simulink model "EfestoRocketEngine_28_04_23"  (R2023a)
settings: Solver=VariableStepAuto  StartTime=0.0  StopTime=50  RelTol=1e-3
libraries: matrix_library x2, shared3dof x1
settings Model: Creator=giuse  LastModifiedBy=mattiasaba
settings DebuggingCC: UnconnectedInputMsg=warning  UnconnectedOutputMsg=warning  UnconnectedLineMsg=warning
settings ModelReferenceCC: EnableRefExpFcnMdlSchedulingChecks=on
settings RTWCC: DLArmComputeVersion=19.05

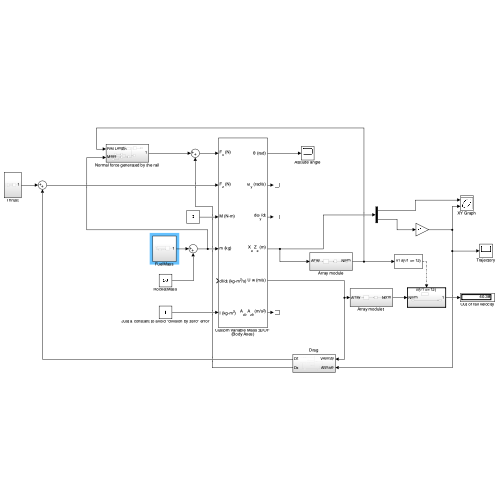
[thumbnail: Simulink's stored preview of the top-level diagram]
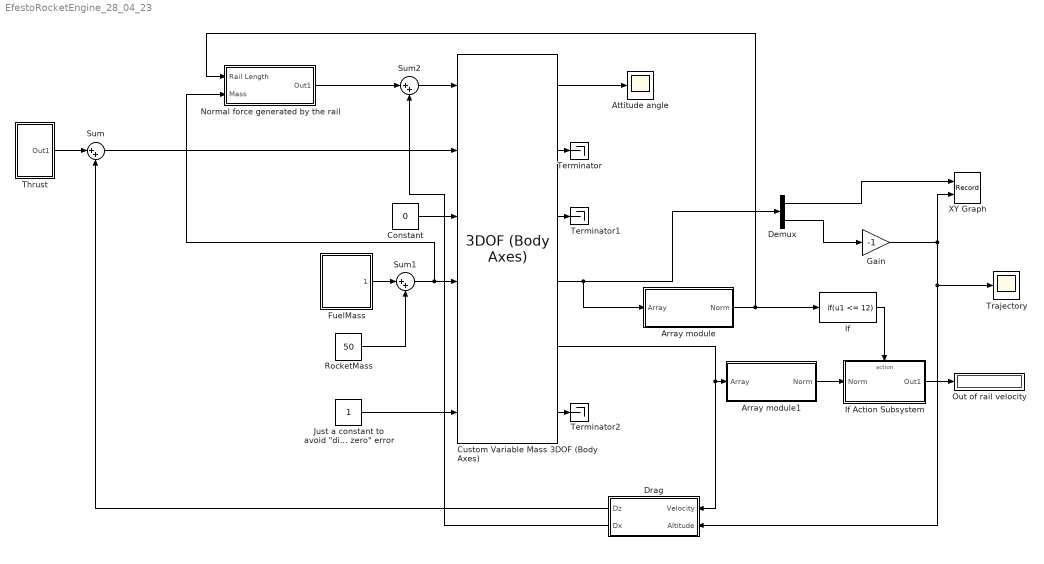
== system EfestoRocketEngine_28_04_23 ==
  Array module : Subsystem
  Array module1 : Subsystem
  Attitude angle : Scope
  Constant : Constant  Value=0
  Custom Variable Mass 3DOF (Body Axes) : shared3dof/3DOF (Body Axes)  units=Metric (MKS)  mtype=Custom Variable  v_ini=0  theta_ini=pi  alpha_ini=0  pos_ini=[0 0]  q_ini=0  mass=1.0  mass_e=0.5  mass_f=3.0  Iyy=1.0  Iyy_e=0.5  Iyy_f=3.0  g_in=Internal  g=9.81  vre_flag=off  abi_flag=off  aMode=0  vel_statename=''  theta_statename=''  pos_statename=''  q_statename=''  mass_statename=''
  Demux : Demux  Outputs=2
  Drag : Subsystem
  FuelMass : Subsystem
  Gain : Gain  Gain=-1
  If : If  IfExpression=u1 <= 12  ShowElse=off
  If Action Subsystem : Subsystem  TreatAsAtomicUnit=on
  "Just a constant to avoid \"division by zero\" error" : Constant
  Normal force generated by the rail : Subsystem
  Out of rail velocity : Display
  RocketMass : Constant  Value=50
  Sum : Sum  Inputs=|++
  Sum1 : Sum  Inputs=|++
  Sum2 : Sum  Inputs=|++
  Terminator : Terminator
  Terminator1 : Terminator
  Terminator2 : Terminator
  Thrust : Subsystem
  Trajectory : Scope
  XY Graph : Record  FileSettingsInternal="{\"entries\":[{\"content\":{\"excelSettings\":{\"content\":{},\"type\":\"Streamout.ExcelSettings\"}},\"type\":\"Streamout.FileSettingStorage\",\"uuid\":\"102b2f02-9d14-4766-8d69-63aa978f5510\"}],\"packageUris\":[\"http://schema.mathworks.com/mf0/streamout_blocks/R2020a\"],\"version\":\"1.0\"}"  Layout=[1 1]  SignalsInternal="{\"entries\":[{\"content\":{\"signals\":[{\"content\":{\"blockPath\":[\"EfestoRocketEngine_28_04_23/XY Graph\"],\"dimensions\":[1],\"domain\":\"EfestoRocketEngine_28_04_23/XY Graph\",\"lineColor\":\"#a2142f\",\"plots\":[1],\"port\":1,\"sid\":[\"\"],\"signalID\":96,\"signalName\":\"Demux:1\"},\"type\":\"RecordBlkView.Signal\",\"uuid\":\"11d17661-1dd1-4241-8cf8-6f9b05c222c4\"},{\"content\":{\"blockPath\":[\"EfestoRocketEngine_28_04_23/XY Graph\"],\"dimensions\":[1],\"domain\":\"EfestoRocketEngine_28_04_23/XY Graph\",\"lineColor\":\"#139fff\",\"plots\":[1],\"port\":2,\"sid\":[\"\"],\"signalID\":100,\"signalName\":\"Gain\"},\"type\":\"RecordBlkView.Signal\",\"uuid\":\"dbca8d71-ba0e-47b5-92a1-924a943d85be\"}]},\"type\":\"RecordBlkView.InputSignals\",\"uuid\":\"7a493edc-8874-4727-801b-36ee9696f784\"}],\"packageUris\":[\"http://schema.mathworks.com/mf0/streamout_blocks/R2020a\"],\"version\":\"1.0\"}"  VisualizationBindings="{\"xyplotplugin\":{\"info\":[{\"series\":[{\"bindingParametersList\":[{\"parameter\":\"X-Axis\",\"signalID\":96,\"signalName\":\"Demux:1\"},{\"parameter\":\"Y-Axis\",\"signalID\":100,\"signalName\":\"Gain\"}],\"seriesID\":31883}],\"subplotID\":1}]}}"  CompatibilityTag=XY  st=-1
  wires:
  Gain/1 -> Drag/2(Altitude), Trajectory/1, XY Graph/2
  Demux/2 -> Gain/1
  Demux/1 -> XY Graph/1
  Custom Variable Mass 3DOF (Body Axes)/4 -> Array module/1(Array), Demux/1
  Custom Variable Mass 3DOF (Body Axes)/5 -> Drag/1(Velocity), Array module1/1(Array)
  Drag/1(Dz) -> Sum/2
  Custom Variable Mass 3DOF (Body Axes)/1 -> Attitude angle/1
  Constant/1 -> Custom Variable Mass 3DOF (Body Axes)/3
  Custom Variable Mass 3DOF (Body Axes)/2 -> Terminator/1
  Custom Variable Mass 3DOF (Body Axes)/3 -> Terminator1/1
  Custom Variable Mass 3DOF (Body Axes)/6 -> Terminator2/1
  RocketMass/1 -> Sum1/2
  "Just a constant to avoid \"division by zero\" error"/1 -> Custom Variable Mass 3DOF (Body Axes)/6
  If/1 -> If Action Subsystem/Action
  If Action Subsystem/1(Out1) -> Out of rail velocity/1
  Sum/1 -> Custom Variable Mass 3DOF (Body Axes)/2
  Sum1/1 -> Normal force generated by the rail/2(Mass), Custom Variable Mass 3DOF (Body Axes)/4
  Array module1/1(Norm) -> If Action Subsystem/1(Norm)
  Array module/1(Norm) -> Normal force generated by the rail/1(Rail Length), If/1
  Normal force generated by the rail/1(Out1) -> Sum2/1
  FuelMass/1(1) -> Sum1/1
  Thrust/1(Out1) -> Sum/1
  Drag/2(Dx) -> Sum2/2
  Sum2/1 -> Custom Variable Mass 3DOF (Body Axes)/1

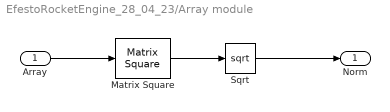
== system EfestoRocketEngine_28_04_23/Array module ==
  Array : Inport
  Matrix Square : matrix_library/Matrix Square  OutMin=[]  OutMax=[]
      settings: LibrarySourceBlock=|
      | simulink/Matrix
      | Operations/Matrix
      | Square
  Sqrt : Sqrt
  Norm : Outport
  wires:
  Array/1 -> Matrix Square/1
  Matrix Square/1 -> Sqrt/1
  Sqrt/1 -> Norm/1

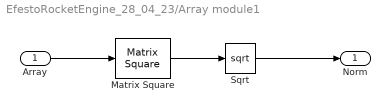
== system EfestoRocketEngine_28_04_23/Array module1 ==
  Array : Inport
  Matrix Square : matrix_library/Matrix Square  OutMin=[]  OutMax=[]
      settings: LibrarySourceBlock=|
      | simulink/Matrix
      | Operations/Matrix
      | Square
  Sqrt : Sqrt
  Norm : Outport
  wires:
  Array/1 -> Matrix Square/1
  Matrix Square/1 -> Sqrt/1
  Sqrt/1 -> Norm/1

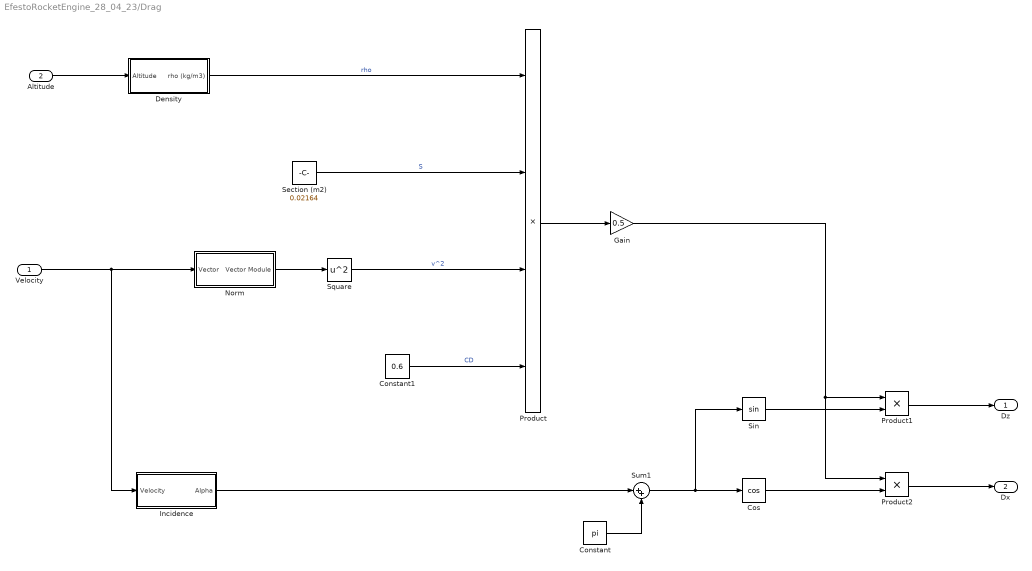
== system EfestoRocketEngine_28_04_23/Drag ==
  Velocity : Inport
  Altitude : Inport  Port=2
  Constant : Constant  Value=pi
  Constant1 : Constant  Value=0.6
  Cos : Trigonometry  Operator=cos
  Density : Subsystem
  Gain : Gain  Gain=0.5
  Incidence : Subsystem
  Norm : Subsystem
  Product : Product  Inputs=4
  Product1 : Product
  Product2 : Product
  Section (m2) : Constant  Value=0.02164
  Sin : Trigonometry
  Square : Math  Operator=square
  Sum1 : Sum  Inputs=|++
  Dz : Outport
  Dx : Outport  Port=2
  wires:
  Velocity/1 -> Incidence/1(Velocity), Norm/1(Vector)
  Altitude/1 -> Density/1(Altitude)
  Incidence/1(Alpha) -> Sum1/1
  Norm/1(Vector Module) -> Square/1
  Density/1(rho (kg/m3)) -> Product/1  "rho"
  Section (m2)/1 -> Product/2  "S"
  Square/1 -> Product/3  "v^2"
  Product/1 -> Gain/1
  Constant1/1 -> Product/4  "CD"
  Constant/1 -> Sum1/2
  Sum1/1 -> Sin/1, Cos/1
  Sin/1 -> Product1/2
  Gain/1 -> Product2/1, Product1/1
  Cos/1 -> Product2/2
  Product2/1 -> Dx/1
  Product1/1 -> Dz/1

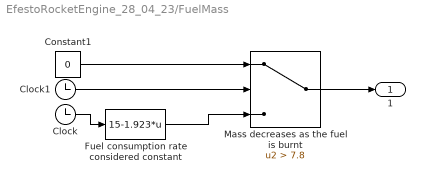
== system EfestoRocketEngine_28_04_23/FuelMass ==
  Clock : Clock
  Clock1 : Clock
  Constant1 : Constant  Value=0
  Fuel consumption rate considered constant : Fcn  Expr=15-1.923*u
  Mass decreases as the fuel is burnt : Switch  Criteria=u2 > Threshold  Threshold=7.8  SaturateOnIntegerOverflow=off  InputSameDT=off
  1 : Outport
  wires:
  Clock/1 -> Fuel consumption rate considered constant/1
  Mass decreases as the fuel is burnt/1 -> 1/1
  Fuel consumption rate considered constant/1 -> Mass decreases as the fuel is burnt/3
  Clock1/1 -> Mass decreases as the fuel is burnt/2
  Constant1/1 -> Mass decreases as the fuel is burnt/1

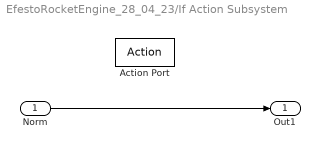
== system EfestoRocketEngine_28_04_23/If Action Subsystem ==
  Norm : Inport
  Action Port : ActionPort  ActionPortLabel=if(u1 <= 12)
  Out1 : Outport
  wires:
  Norm/1 -> Out1/1

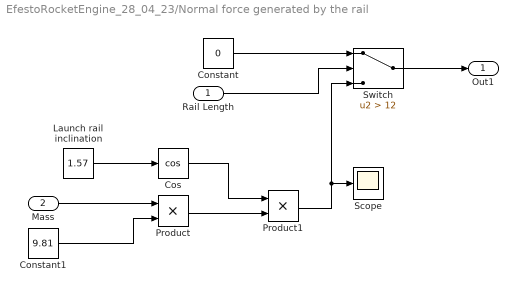
== system EfestoRocketEngine_28_04_23/Normal force generated by the rail ==
  Rail Length : Inport
  Mass : Inport  Port=2
  Constant : Constant  Value=0
  Constant1 : Constant  Value=9.81
  Cos : Trigonometry  Operator=cos
  "Launch rail inclination " : Constant  Value=1.57
  Product : Product
  Product1 : Product
  Scope : Scope
  Switch : Switch  Criteria=u2 > Threshold  Threshold=12  SaturateOnIntegerOverflow=off  InputSameDT=off
  Out1 : Outport
  wires:
  Rail Length/1 -> Switch/2
  Constant/1 -> Switch/1
  Mass/1 -> Product/1
  Constant1/1 -> Product/2
  Product/1 -> Product1/2
  Switch/1 -> Out1/1
  Cos/1 -> Product1/1
  Product1/1 -> Scope/1, Switch/3
  "Launch rail inclination "/1 -> Cos/1

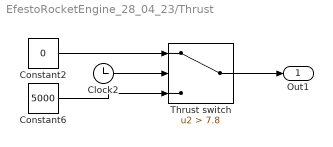
== system EfestoRocketEngine_28_04_23/Thrust ==
  Clock2 : Clock
  Constant2 : Constant  Value=0
  Constant6 : Constant  Value=5000
  Thrust switch : Switch  Criteria=u2 > Threshold  Threshold=7.8  SaturateOnIntegerOverflow=off  InputSameDT=off
  Out1 : Outport
  wires:
  Clock2/1 -> Thrust switch/2
  Thrust switch/1 -> Out1/1
  Constant2/1 -> Thrust switch/1
  Constant6/1 -> Thrust switch/3

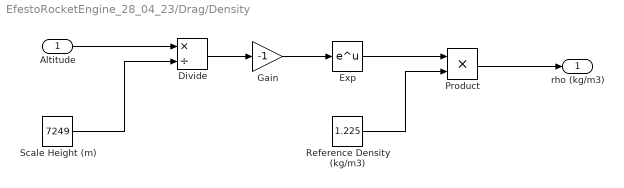
== system EfestoRocketEngine_28_04_23/Drag/Density ==
  Altitude : Inport
  Divide : Product  Inputs=*/
  Exp : Math
  Gain : Gain  Gain=-1
  Product : Product
  Reference Density (kg/m3) : Constant  Value=1.225
  Scale Height (m) : Constant  Value=7249
  rho (kg/m3) : Outport
  wires:
  Altitude/1 -> Divide/1
  Scale Height (m)/1 -> Divide/2
  Divide/1 -> Gain/1
  Gain/1 -> Exp/1
  Exp/1 -> Product/1
  Reference Density (kg/m3)/1 -> Product/2
  Product/1 -> rho (kg/m3)/1

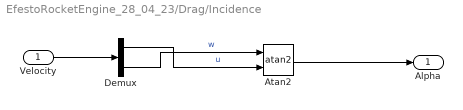
== system EfestoRocketEngine_28_04_23/Drag/Incidence ==
  Velocity : Inport
  Atan2 : Trigonometry  Operator=atan2
  Demux : Demux  Outputs=2
  Alpha : Outport
  wires:
  Velocity/1 -> Demux/1
  Demux/2 -> Atan2/1  "w"
  Demux/1 -> Atan2/2  "u"
  Atan2/1 -> Alpha/1

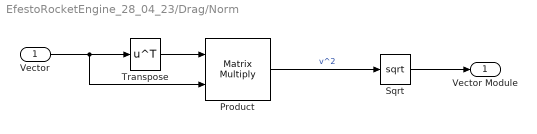
== system EfestoRocketEngine_28_04_23/Drag/Norm ==
  Vector : Inport
  Product : Product  Multiplication=Matrix(*)
  Sqrt : Sqrt
  Transpose : Math  Operator=transpose
  Vector Module : Outport
  wires:
  Vector/1 -> Product/2, Transpose/1
  Product/1 -> Sqrt/1  "v^2"
  Sqrt/1 -> Vector Module/1
  Transpose/1 -> Product/1
